simulink library "sm_robot_6legs_4bar_lib"  (R2026a)
settings: Solver=VariableStepAuto
undefined symbols (not defined in the file): frame_wid, link_h, link_th, Local, X, Z
libraries: Parts_Lib x57, sm_lib x15
Description:
  | Copyright 2018-2026 The MathWorks, Inc.
settings Model: Creator=smiller  LastModifiedBy=smiller
settings DebuggingCC: PregeneratedLibrarySubsystemCodeDiagnostic=none

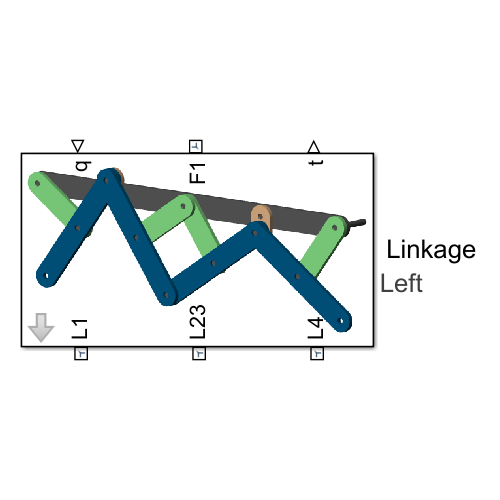
[thumbnail: Simulink's stored preview of the top-level diagram]
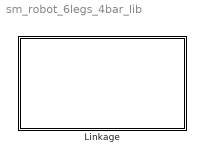
== system sm_robot_6legs_4bar_lib ==
  Linkage : Subsystem  mask(Leg Mechanism and Frame){popup_LorR=Left}
      mask prompts: popup_LorR "Side"
      mask help: Two connected four-bar linkages form three legs for one side of a 6-legged robot. Set the parameter below to select the side of the robot. Dimensions and other parameters are defined using variables in the MATLAB Workspace.
      mask init:
      | f    = Simulink.FindOptions('FollowLinks',1,'LookUnderMasks','all','regexp',1);
      | temp_rod_pth = Simulink.findBlocks(bdroot,'ReferenceBlock','.*Rod','popup_zori','.*',f);
      | 
      | if(popup_LorR == 1)
      |     rod_setting = 0;
      |     set_param([gcb '/Revolute Cam L12'],'PositionTargetValue','270');
      |     set_param([gcb '/Revolute Cam L34'],'PositionTargetValue','90');
      | else
      |     rod_setting = 1;
      |     set_param([gcb '/Revolute Cam L12'],'PositionTargetValue','90');
      |     set_param([gcb '/Revolute Cam L34'],'PositionTargetValue','270');
      | end
      | 
      | for temp_rod_i = 1:length(temp_rod_pth)
      |     set_param(temp_rod_pth(temp_rod_i),'popup_zori',rod_setting);
      | end
      settings: AttributesFormatString=%<popup_LorR>
      mask TypeOptions popup_LorR: Left | Right
      mask Display:
      | if(strcmpi(get_param(gcb,'popup_LorR'),'Left'))
      |     image('sm_robot_6legs_4bar_Linkage_Left_IMAGE.png');
      | else
      |     image('sm_robot_6legs_4bar_Linkage_Right_IMAGE.png');
      | end

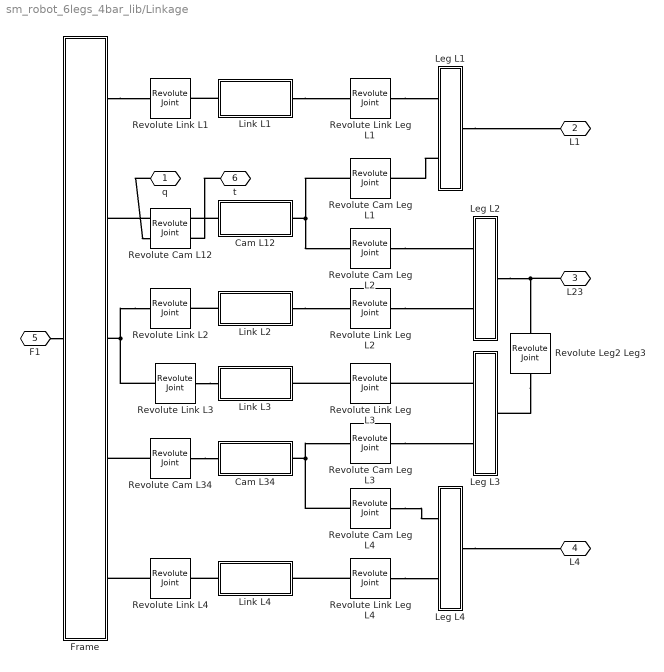
== system sm_robot_6legs_4bar_lib/Linkage ==
  Cam L12 : Subsystem
  Cam L34 : Subsystem
  Frame : Subsystem
  Leg L1 : Subsystem
  Leg L2 : Subsystem
  Leg L3 : Subsystem
  Leg L4 : Subsystem
  Link L1 : Subsystem
  Link L2 : Subsystem
  Link L3 : Subsystem
  Link L4 : Subsystem
  Revolute Leg2 Leg3 : sm_lib/Joints/Revolute Joint  JointMode=Normal  CompositeWrenchDir=FollowerOnBase  CompositeWrenchFrame=BaseFrame  SenseConstraintForce=off  SenseConstraintTorque=off  SenseTotalForce=off  SenseTotalTorque=off  PositionTargetSpecify=on  PositionTargetPriority=Low  PositionTargetValue=-90  PositionTargetValueUnits=deg  VelocityTargetSpecify=off  VelocityTargetPriority=High  VelocityTargetValue=0  VelocityTargetValueUnits=deg/s  EquilibriumPosition=0  EquilibriumPositionUnits=deg  SpringStiffness=0  SpringStiffnessUnits=N*m/deg  DampingCoefficient=0  DampingCoefficientUnits=N*m/(deg/s)  LowerLimitSpecify=off  LowerLimitBound=-90  LowerLimitBoundUnits=deg  LowerLimitStiffness=1e4  LowerLimitStiffnessUnits=N*m/deg  LowerLimitDamping=10  LowerLimitDampingUnits=N*m/(deg/s)  LowerLimitTransitionRegionWidth=0.1  LowerLimitTransitionRegionWidthUnits=deg  UpperLimitSpecify=off  UpperLimitBound=90  UpperLimitBoundUnits=deg  UpperLimitStiffness=1e4  UpperLimitStiffnessUnits=N*m/deg  UpperLimitDamping=10  UpperLimitDampingUnits=N*m/(deg/s)  UpperLimitTransitionRegionWidth=0.1  UpperLimitTransitionRegionWidthUnits=deg  TorqueActuationMode=NoTorque  MotionActuationMode=ComputedMotion  SensePosition=off  SenseVelocity=off  SenseAcceleration=off  SenseTorqueForce=off  SenseLowerLimitTorqueForce=off  SenseUpperLimitTorqueForce=off
      settings: AttributesFormatString=t0: %<PositionTargetValue> %<PositionTargetValueUnits>, %<PositionTargetPriority>
  Revolute Cam L12 : sm_lib/Joints/Revolute Joint  JointMode=Normal  CompositeWrenchDir=FollowerOnBase  CompositeWrenchFrame=BaseFrame  SenseConstraintForce=off  SenseConstraintTorque=off  SenseTotalForce=off  SenseTotalTorque=off  PositionTargetSpecify=on  PositionTargetPriority=High  PositionTargetValue=270  PositionTargetValueUnits=deg  VelocityTargetSpecify=off  VelocityTargetPriority=High  VelocityTargetValue=0  VelocityTargetValueUnits=deg/s  EquilibriumPosition=0  EquilibriumPositionUnits=deg  SpringStiffness=0  SpringStiffnessUnits=N*m/deg  DampingCoefficient=0.001  DampingCoefficientUnits=N*m/(deg/s)  LowerLimitSpecify=off  LowerLimitBound=-90  LowerLimitBoundUnits=deg  LowerLimitStiffness=1e4  LowerLimitStiffnessUnits=N*m/deg  LowerLimitDamping=10  LowerLimitDampingUnits=N*m/(deg/s)  LowerLimitTransitionRegionWidth=0.1  LowerLimitTransitionRegionWidthUnits=deg  UpperLimitSpecify=off  UpperLimitBound=90  UpperLimitBoundUnits=deg  UpperLimitStiffness=1e4  UpperLimitStiffnessUnits=N*m/deg  UpperLimitDamping=10  UpperLimitDampingUnits=N*m/(deg/s)  UpperLimitTransitionRegionWidth=0.1  UpperLimitTransitionRegionWidthUnits=deg  TorqueActuationMode=ComputedTorque  MotionActuationMode=InputMotion  SensePosition=off  SenseVelocity=off  SenseAcceleration=off  SenseTorqueForce=on  SenseLowerLimitTorqueForce=off  SenseUpperLimitTorqueForce=off
      settings: AttributesFormatString=t0: %<PositionTargetValue> %<PositionTargetValueUnits>, %<PositionTargetPriority>
  Revolute Cam L34 : sm_lib/Joints/Revolute Joint  JointMode=Normal  CompositeWrenchDir=FollowerOnBase  CompositeWrenchFrame=BaseFrame  SenseConstraintForce=off  SenseConstraintTorque=off  SenseTotalForce=off  SenseTotalTorque=off  PositionTargetSpecify=on  PositionTargetPriority=Low  PositionTargetValue=90  PositionTargetValueUnits=deg  VelocityTargetSpecify=off  VelocityTargetPriority=High  VelocityTargetValue=0  VelocityTargetValueUnits=deg/s  EquilibriumPosition=0  EquilibriumPositionUnits=deg  SpringStiffness=0  SpringStiffnessUnits=N*m/deg  DampingCoefficient=0  DampingCoefficientUnits=N*m/(deg/s)  LowerLimitSpecify=off  LowerLimitBound=-90  LowerLimitBoundUnits=deg  LowerLimitStiffness=1e4  LowerLimitStiffnessUnits=N*m/deg  LowerLimitDamping=10  LowerLimitDampingUnits=N*m/(deg/s)  LowerLimitTransitionRegionWidth=0.1  LowerLimitTransitionRegionWidthUnits=deg  UpperLimitSpecify=off  UpperLimitBound=90  UpperLimitBoundUnits=deg  UpperLimitStiffness=1e4  UpperLimitStiffnessUnits=N*m/deg  UpperLimitDamping=10  UpperLimitDampingUnits=N*m/(deg/s)  UpperLimitTransitionRegionWidth=0.1  UpperLimitTransitionRegionWidthUnits=deg  TorqueActuationMode=NoTorque  MotionActuationMode=ComputedMotion  SensePosition=off  SenseVelocity=off  SenseAcceleration=off  SenseTorqueForce=off  SenseLowerLimitTorqueForce=off  SenseUpperLimitTorqueForce=off
      settings: AttributesFormatString=t0: %<PositionTargetValue> %<PositionTargetValueUnits>, %<PositionTargetPriority>
  Revolute Cam Leg L1 : sm_lib/Joints/Revolute Joint  JointMode=Normal  CompositeWrenchDir=FollowerOnBase  CompositeWrenchFrame=BaseFrame  SenseConstraintForce=off  SenseConstraintTorque=off  SenseTotalForce=off  SenseTotalTorque=off  PositionTargetSpecify=off  PositionTargetPriority=Low  PositionTargetValue=135  PositionTargetValueUnits=deg  VelocityTargetSpecify=off  VelocityTargetPriority=High  VelocityTargetValue=0  VelocityTargetValueUnits=deg/s  EquilibriumPosition=0  EquilibriumPositionUnits=deg  SpringStiffness=0  SpringStiffnessUnits=N*m/deg  DampingCoefficient=0  DampingCoefficientUnits=N*m/(deg/s)  LowerLimitSpecify=off  LowerLimitBound=-90  LowerLimitBoundUnits=deg  LowerLimitStiffness=1e4  LowerLimitStiffnessUnits=N*m/deg  LowerLimitDamping=10  LowerLimitDampingUnits=N*m/(deg/s)  LowerLimitTransitionRegionWidth=0.1  LowerLimitTransitionRegionWidthUnits=deg  UpperLimitSpecify=off  UpperLimitBound=90  UpperLimitBoundUnits=deg  UpperLimitStiffness=1e4  UpperLimitStiffnessUnits=N*m/deg  UpperLimitDamping=10  UpperLimitDampingUnits=N*m/(deg/s)  UpperLimitTransitionRegionWidth=0.1  UpperLimitTransitionRegionWidthUnits=deg  TorqueActuationMode=NoTorque  MotionActuationMode=ComputedMotion  SensePosition=off  SenseVelocity=off  SenseAcceleration=off  SenseTorqueForce=off  SenseLowerLimitTorqueForce=off  SenseUpperLimitTorqueForce=off
  Revolute Cam Leg L2 : sm_lib/Joints/Revolute Joint  JointMode=Normal  CompositeWrenchDir=FollowerOnBase  CompositeWrenchFrame=BaseFrame  SenseConstraintForce=off  SenseConstraintTorque=off  SenseTotalForce=off  SenseTotalTorque=off  PositionTargetSpecify=off  PositionTargetPriority=Low  PositionTargetValue=-135  PositionTargetValueUnits=deg  VelocityTargetSpecify=off  VelocityTargetPriority=High  VelocityTargetValue=0  VelocityTargetValueUnits=deg/s  EquilibriumPosition=0  EquilibriumPositionUnits=deg  SpringStiffness=0  SpringStiffnessUnits=N*m/deg  DampingCoefficient=0  DampingCoefficientUnits=N*m/(deg/s)  LowerLimitSpecify=off  LowerLimitBound=-90  LowerLimitBoundUnits=deg  LowerLimitStiffness=1e4  LowerLimitStiffnessUnits=N*m/deg  LowerLimitDamping=10  LowerLimitDampingUnits=N*m/(deg/s)  LowerLimitTransitionRegionWidth=0.1  LowerLimitTransitionRegionWidthUnits=deg  UpperLimitSpecify=off  UpperLimitBound=90  UpperLimitBoundUnits=deg  UpperLimitStiffness=1e4  UpperLimitStiffnessUnits=N*m/deg  UpperLimitDamping=10  UpperLimitDampingUnits=N*m/(deg/s)  UpperLimitTransitionRegionWidth=0.1  UpperLimitTransitionRegionWidthUnits=deg  TorqueActuationMode=NoTorque  MotionActuationMode=ComputedMotion  SensePosition=off  SenseVelocity=off  SenseAcceleration=off  SenseTorqueForce=off  SenseLowerLimitTorqueForce=off  SenseUpperLimitTorqueForce=off
  Revolute Cam Leg L3 : sm_lib/Joints/Revolute Joint  JointMode=Normal  CompositeWrenchDir=FollowerOnBase  CompositeWrenchFrame=BaseFrame  SenseConstraintForce=off  SenseConstraintTorque=off  SenseTotalForce=off  SenseTotalTorque=off  PositionTargetSpecify=off  PositionTargetPriority=High  PositionTargetValue=0  PositionTargetValueUnits=deg  VelocityTargetSpecify=off  VelocityTargetPriority=High  VelocityTargetValue=0  VelocityTargetValueUnits=deg/s  EquilibriumPosition=0  EquilibriumPositionUnits=deg  SpringStiffness=0  SpringStiffnessUnits=N*m/deg  DampingCoefficient=0  DampingCoefficientUnits=N*m/(deg/s)  LowerLimitSpecify=off  LowerLimitBound=-90  LowerLimitBoundUnits=deg  LowerLimitStiffness=1e4  LowerLimitStiffnessUnits=N*m/deg  LowerLimitDamping=10  LowerLimitDampingUnits=N*m/(deg/s)  LowerLimitTransitionRegionWidth=0.1  LowerLimitTransitionRegionWidthUnits=deg  UpperLimitSpecify=off  UpperLimitBound=90  UpperLimitBoundUnits=deg  UpperLimitStiffness=1e4  UpperLimitStiffnessUnits=N*m/deg  UpperLimitDamping=10  UpperLimitDampingUnits=N*m/(deg/s)  UpperLimitTransitionRegionWidth=0.1  UpperLimitTransitionRegionWidthUnits=deg  TorqueActuationMode=NoTorque  MotionActuationMode=ComputedMotion  SensePosition=off  SenseVelocity=off  SenseAcceleration=off  SenseTorqueForce=off  SenseLowerLimitTorqueForce=off  SenseUpperLimitTorqueForce=off
  Revolute Cam Leg L4 : sm_lib/Joints/Revolute Joint  JointMode=Normal  CompositeWrenchDir=FollowerOnBase  CompositeWrenchFrame=BaseFrame  SenseConstraintForce=off  SenseConstraintTorque=off  SenseTotalForce=off  SenseTotalTorque=off  PositionTargetSpecify=off  PositionTargetPriority=High  PositionTargetValue=0  PositionTargetValueUnits=deg  VelocityTargetSpecify=off  VelocityTargetPriority=High  VelocityTargetValue=0  VelocityTargetValueUnits=deg/s  EquilibriumPosition=0  EquilibriumPositionUnits=deg  SpringStiffness=0  SpringStiffnessUnits=N*m/deg  DampingCoefficient=0  DampingCoefficientUnits=N*m/(deg/s)  LowerLimitSpecify=off  LowerLimitBound=-90  LowerLimitBoundUnits=deg  LowerLimitStiffness=1e4  LowerLimitStiffnessUnits=N*m/deg  LowerLimitDamping=10  LowerLimitDampingUnits=N*m/(deg/s)  LowerLimitTransitionRegionWidth=0.1  LowerLimitTransitionRegionWidthUnits=deg  UpperLimitSpecify=off  UpperLimitBound=90  UpperLimitBoundUnits=deg  UpperLimitStiffness=1e4  UpperLimitStiffnessUnits=N*m/deg  UpperLimitDamping=10  UpperLimitDampingUnits=N*m/(deg/s)  UpperLimitTransitionRegionWidth=0.1  UpperLimitTransitionRegionWidthUnits=deg  TorqueActuationMode=NoTorque  MotionActuationMode=ComputedMotion  SensePosition=off  SenseVelocity=off  SenseAcceleration=off  SenseTorqueForce=off  SenseLowerLimitTorqueForce=off  SenseUpperLimitTorqueForce=off
  Revolute Link L1 : sm_lib/Joints/Revolute Joint  JointMode=Normal  CompositeWrenchDir=FollowerOnBase  CompositeWrenchFrame=BaseFrame  SenseConstraintForce=off  SenseConstraintTorque=off  SenseTotalForce=off  SenseTotalTorque=off  PositionTargetSpecify=on  PositionTargetPriority=Low  PositionTargetValue=-90  PositionTargetValueUnits=deg  VelocityTargetSpecify=off  VelocityTargetPriority=High  VelocityTargetValue=0  VelocityTargetValueUnits=deg/s  EquilibriumPosition=0  EquilibriumPositionUnits=deg  SpringStiffness=0  SpringStiffnessUnits=N*m/deg  DampingCoefficient=0  DampingCoefficientUnits=N*m/(deg/s)  LowerLimitSpecify=off  LowerLimitBound=-90  LowerLimitBoundUnits=deg  LowerLimitStiffness=1e4  LowerLimitStiffnessUnits=N*m/deg  LowerLimitDamping=10  LowerLimitDampingUnits=N*m/(deg/s)  LowerLimitTransitionRegionWidth=0.1  LowerLimitTransitionRegionWidthUnits=deg  UpperLimitSpecify=off  UpperLimitBound=90  UpperLimitBoundUnits=deg  UpperLimitStiffness=1e4  UpperLimitStiffnessUnits=N*m/deg  UpperLimitDamping=10  UpperLimitDampingUnits=N*m/(deg/s)  UpperLimitTransitionRegionWidth=0.1  UpperLimitTransitionRegionWidthUnits=deg  TorqueActuationMode=NoTorque  MotionActuationMode=ComputedMotion  SensePosition=off  SenseVelocity=off  SenseAcceleration=off  SenseTorqueForce=off  SenseLowerLimitTorqueForce=off  SenseUpperLimitTorqueForce=off
      settings: AttributesFormatString=t0: %<PositionTargetValue> %<PositionTargetValueUnits>, %<PositionTargetPriority>
  Revolute Link L2 : sm_lib/Joints/Revolute Joint  JointMode=Normal  CompositeWrenchDir=FollowerOnBase  CompositeWrenchFrame=BaseFrame  SenseConstraintForce=off  SenseConstraintTorque=off  SenseTotalForce=off  SenseTotalTorque=off  PositionTargetSpecify=off  PositionTargetPriority=High  PositionTargetValue=0  PositionTargetValueUnits=deg  VelocityTargetSpecify=off  VelocityTargetPriority=High  VelocityTargetValue=0  VelocityTargetValueUnits=deg/s  EquilibriumPosition=0  EquilibriumPositionUnits=deg  SpringStiffness=0  SpringStiffnessUnits=N*m/deg  DampingCoefficient=0  DampingCoefficientUnits=N*m/(deg/s)  LowerLimitSpecify=off  LowerLimitBound=-90  LowerLimitBoundUnits=deg  LowerLimitStiffness=1e4  LowerLimitStiffnessUnits=N*m/deg  LowerLimitDamping=10  LowerLimitDampingUnits=N*m/(deg/s)  LowerLimitTransitionRegionWidth=0.1  LowerLimitTransitionRegionWidthUnits=deg  UpperLimitSpecify=off  UpperLimitBound=90  UpperLimitBoundUnits=deg  UpperLimitStiffness=1e4  UpperLimitStiffnessUnits=N*m/deg  UpperLimitDamping=10  UpperLimitDampingUnits=N*m/(deg/s)  UpperLimitTransitionRegionWidth=0.1  UpperLimitTransitionRegionWidthUnits=deg  TorqueActuationMode=NoTorque  MotionActuationMode=ComputedMotion  SensePosition=off  SenseVelocity=off  SenseAcceleration=off  SenseTorqueForce=off  SenseLowerLimitTorqueForce=off  SenseUpperLimitTorqueForce=off
  Revolute Link L3 : sm_lib/Joints/Revolute Joint  JointMode=Normal  CompositeWrenchDir=FollowerOnBase  CompositeWrenchFrame=BaseFrame  SenseConstraintForce=off  SenseConstraintTorque=off  SenseTotalForce=off  SenseTotalTorque=off  PositionTargetSpecify=off  PositionTargetPriority=Low  PositionTargetValue=-135  PositionTargetValueUnits=deg  VelocityTargetSpecify=off  VelocityTargetPriority=High  VelocityTargetValue=0  VelocityTargetValueUnits=deg/s  EquilibriumPosition=0  EquilibriumPositionUnits=deg  SpringStiffness=0  SpringStiffnessUnits=N*m/deg  DampingCoefficient=0  DampingCoefficientUnits=N*m/(deg/s)  LowerLimitSpecify=off  LowerLimitBound=-90  LowerLimitBoundUnits=deg  LowerLimitStiffness=1e4  LowerLimitStiffnessUnits=N*m/deg  LowerLimitDamping=10  LowerLimitDampingUnits=N*m/(deg/s)  LowerLimitTransitionRegionWidth=0.1  LowerLimitTransitionRegionWidthUnits=deg  UpperLimitSpecify=off  UpperLimitBound=90  UpperLimitBoundUnits=deg  UpperLimitStiffness=1e4  UpperLimitStiffnessUnits=N*m/deg  UpperLimitDamping=10  UpperLimitDampingUnits=N*m/(deg/s)  UpperLimitTransitionRegionWidth=0.1  UpperLimitTransitionRegionWidthUnits=deg  TorqueActuationMode=NoTorque  MotionActuationMode=ComputedMotion  SensePosition=off  SenseVelocity=off  SenseAcceleration=off  SenseTorqueForce=off  SenseLowerLimitTorqueForce=off  SenseUpperLimitTorqueForce=off
  Revolute Link L4 : sm_lib/Joints/Revolute Joint  JointMode=Normal  CompositeWrenchDir=FollowerOnBase  CompositeWrenchFrame=BaseFrame  SenseConstraintForce=off  SenseConstraintTorque=off  SenseTotalForce=off  SenseTotalTorque=off  PositionTargetSpecify=on  PositionTargetPriority=Low  PositionTargetValue=-90  PositionTargetValueUnits=deg  VelocityTargetSpecify=off  VelocityTargetPriority=High  VelocityTargetValue=0  VelocityTargetValueUnits=deg/s  EquilibriumPosition=0  EquilibriumPositionUnits=deg  SpringStiffness=0  SpringStiffnessUnits=N*m/deg  DampingCoefficient=0  DampingCoefficientUnits=N*m/(deg/s)  LowerLimitSpecify=off  LowerLimitBound=-90  LowerLimitBoundUnits=deg  LowerLimitStiffness=1e4  LowerLimitStiffnessUnits=N*m/deg  LowerLimitDamping=10  LowerLimitDampingUnits=N*m/(deg/s)  LowerLimitTransitionRegionWidth=0.1  LowerLimitTransitionRegionWidthUnits=deg  UpperLimitSpecify=off  UpperLimitBound=90  UpperLimitBoundUnits=deg  UpperLimitStiffness=1e4  UpperLimitStiffnessUnits=N*m/deg  UpperLimitDamping=10  UpperLimitDampingUnits=N*m/(deg/s)  UpperLimitTransitionRegionWidth=0.1  UpperLimitTransitionRegionWidthUnits=deg  TorqueActuationMode=NoTorque  MotionActuationMode=ComputedMotion  SensePosition=off  SenseVelocity=off  SenseAcceleration=off  SenseTorqueForce=off  SenseLowerLimitTorqueForce=off  SenseUpperLimitTorqueForce=off
      settings: AttributesFormatString=t0: %<PositionTargetValue> %<PositionTargetValueUnits>, %<PositionTargetPriority>
  Revolute Link Leg L{1..4} (4 alike) : sm_lib/Joints/Revolute Joint  JointMode=Normal  CompositeWrenchDir=FollowerOnBase  CompositeWrenchFrame=BaseFrame  SenseConstraintForce=off  SenseConstraintTorque=off  SenseTotalForce=off  SenseTotalTorque=off  PositionTargetSpecify=off  PositionTargetPriority=High  PositionTargetValue=0  PositionTargetValueUnits=deg  VelocityTargetSpecify=off  VelocityTargetPriority=High  VelocityTargetValue=0  VelocityTargetValueUnits=deg/s  EquilibriumPosition=0  EquilibriumPositionUnits=deg  SpringStiffness=0  SpringStiffnessUnits=N*m/deg  DampingCoefficient=0  DampingCoefficientUnits=N*m/(deg/s)  LowerLimitSpecify=off  LowerLimitBound=-90  LowerLimitBoundUnits=deg  LowerLimitStiffness=1e4  LowerLimitStiffnessUnits=N*m/deg  LowerLimitDamping=10  LowerLimitDampingUnits=N*m/(deg/s)  LowerLimitTransitionRegionWidth=0.1  LowerLimitTransitionRegionWidthUnits=deg  UpperLimitSpecify=off  UpperLimitBound=90  UpperLimitBoundUnits=deg  UpperLimitStiffness=1e4  UpperLimitStiffnessUnits=N*m/deg  UpperLimitDamping=10  UpperLimitDampingUnits=N*m/(deg/s)  UpperLimitTransitionRegionWidth=0.1  UpperLimitTransitionRegionWidthUnits=deg  TorqueActuationMode=NoTorque  MotionActuationMode=ComputedMotion  SensePosition=off  SenseVelocity=off  SenseAcceleration=off  SenseTorqueForce=off  SenseLowerLimitTorqueForce=off  SenseUpperLimitTorqueForce=off
  q : PMIOPort  Side=Left
  L1 : PMIOPort  Port=2  Side=Right
  L23 : PMIOPort  Port=3  Side=Right
  L4 : PMIOPort  Port=4  Side=Right
  F1 : PMIOPort  Port=5  Side=Left
  t : PMIOPort  Port=6  Side=Left
  connections:
  F1/RConn1 -- Frame/RConn1
  Cam L12/RConn1 -- Revolute Cam L12/RConn1
  Leg L4/RConn1 -- L4/RConn1
  Leg L1/LConn2 -- Revolute Cam Leg L1/RConn1
  Leg L2/RConn1 -- L23/RConn1 -- Revolute Leg2 Leg3/LConn1
  Link L2/RConn1 -- Revolute Link Leg L2/RConn1
  Revolute Link L2/LConn1 -- Frame/LConn3 -- Revolute Link L3/LConn1
  Revolute Cam Leg L4/LConn1 -- Revolute Cam Leg L3/LConn1 -- Cam L34/RConn1
  Revolute Leg2 Leg3/RConn1 -- Leg L3/RConn1
  Leg L3/LConn1 -- Revolute Link Leg L3/RConn1
  Revolute Cam L34/RConn1 -- Cam L34/LConn1
  Link L4/LConn1 -- Revolute Link L4/RConn1
  Frame/LConn1 -- Revolute Link L1/LConn1
  Revolute Link Leg L2/LConn1 -- Leg L2/LConn2
  Revolute Cam L12/LConn1 -- Frame/LConn2
  Revolute Cam Leg L2/RConn1 -- Leg L2/LConn1
  Revolute Cam L34/LConn1 -- Frame/LConn4
  Revolute Cam Leg L3/RConn1 -- Leg L3/LConn2
  Revolute Cam Leg L4/RConn1 -- Leg L4/LConn1
  Revolute Link Leg L4/RConn1 -- Leg L4/LConn2
  Revolute Link Leg L3/LConn1 -- Link L3/LConn1
  Link L2/LConn1 -- Revolute Link L2/RConn1
  Link L1/LConn1 -- Revolute Link Leg L1/LConn1
  Cam L12/LConn1 -- Revolute Cam Leg L2/LConn1 -- Revolute Cam Leg L1/LConn1
  Revolute Link Leg L4/LConn1 -- Link L4/RConn1
  Revolute Link Leg L1/RConn1 -- Leg L1/LConn1
  Revolute Link L4/LConn1 -- Frame/LConn5
  Link L1/RConn1 -- Revolute Link L1/RConn1
  Leg L1/RConn1 -- L1/RConn1
  q/RConn1 -- Revolute Cam L12/LConn2
  Revolute Link L3/RConn1 -- Link L3/RConn1
  t/RConn1 -- Revolute Cam L12/RConn2

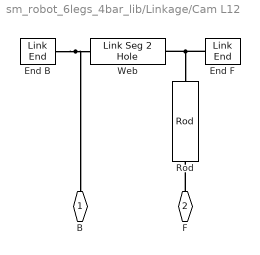
== system sm_robot_6legs_4bar_lib/Linkage/Cam L12 ==
  End B : Parts_Lib/Link End  circ_radout=link_h/2  circ_radin=rad_hole  popup_holelr=-X  deg_1=90  deg_2=270  circ_len=link_th  circ_rho=part_rho  circ_color=cam_clr  circ_opc=1
  End F : Parts_Lib/Link End  circ_radout=link_h/2  circ_radin=rad_hole  popup_holelr=+X  deg_1=-90  deg_2=90  circ_len=link_th  circ_rho=part_rho  circ_color=cam_clr  circ_opc=1
  Rod : Parts_Lib/Rod  rod_rad=rad_hole  rod_len=link_th  rod_rho=part_rho  rod_color=pin_clr  popup_zori=Local +Z  popup_markings=None  mark_radius_range=[0.5 1.01]  mark_length_range=1.005  mark_angle_range=30  mark_color=[1 1 1]
  Web : Parts_Lib/Link Seg 2 Hole  link_len=cam_l  link_width=link_h  link_radh=rad_hole  link_thickness=link_th  link_rho=part_rho  link_color=cam_clr  link_opc=1
  B : PMIOPort  Side=Right
  F : PMIOPort  Port=2  Side=Left
  connections:
  End B/LConn1 -- B/RConn1 -- Web/LConn1
  End F/LConn1 -- Web/RConn1 -- Rod/RConn1
  F/RConn1 -- Rod/LConn1

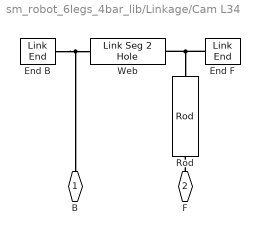
== system sm_robot_6legs_4bar_lib/Linkage/Cam L34 ==
  End B : Parts_Lib/Link End  circ_radout=link_h/2  circ_radin=rad_hole  popup_holelr=-X  deg_1=90  deg_2=270  circ_len=link_th  circ_rho=part_rho  circ_color=cam_clr  circ_opc=1
  End F : Parts_Lib/Link End  circ_radout=link_h/2  circ_radin=rad_hole  popup_holelr=+X  deg_1=-90  deg_2=90  circ_len=link_th  circ_rho=part_rho  circ_color=cam_clr  circ_opc=1
  Rod : Parts_Lib/Rod  rod_rad=rad_hole  rod_len=link_th  rod_rho=part_rho  rod_color=pin_clr  popup_zori=Local +Z  popup_markings=None  mark_radius_range=[0.5 1.01]  mark_length_range=1.005  mark_angle_range=30  mark_color=[1 1 1]
  Web : Parts_Lib/Link Seg 2 Hole  link_len=cam_l  link_width=link_h  link_radh=rad_hole  link_thickness=link_th  link_rho=part_rho  link_color=cam_clr  link_opc=1
  B : PMIOPort  Side=Left
  F : PMIOPort  Port=2  Side=Right
  connections:
  End F/LConn1 -- Web/RConn1 -- Rod/RConn1
  F/RConn1 -- Rod/LConn1
  Web/LConn1 -- End B/LConn1 -- B/RConn1

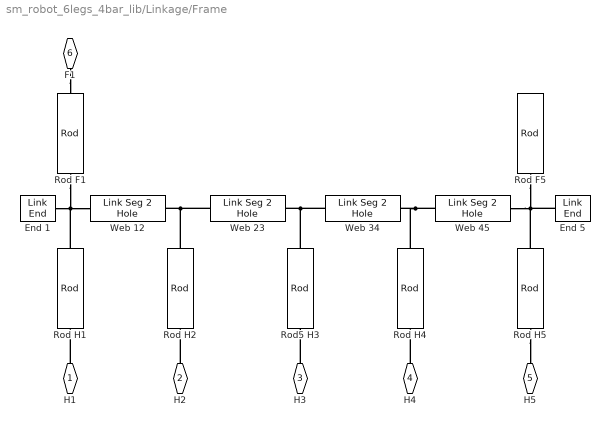
== system sm_robot_6legs_4bar_lib/Linkage/Frame ==
  End 1 : Parts_Lib/Link End  circ_radout=link_h/2  circ_radin=rad_hole  popup_holelr=-X  deg_1=90  deg_2=270  circ_len=link_th  circ_rho=part_rho  circ_color=fra_clr  circ_opc=1
  End 5 : Parts_Lib/Link End  circ_radout=link_h/2  circ_radin=rad_hole  popup_holelr=+X  deg_1=-90  deg_2=90  circ_len=link_th  circ_rho=part_rho  circ_color=fra_clr  circ_opc=1
  Rod F1 : Parts_Lib/Rod  rod_rad=rad_hole  rod_len=frame_wid/2  rod_rho=part_rho  rod_color=pin_clr  popup_zori=Local +Z  popup_markings=None  mark_radius_range=[0.5 1.01]  mark_length_range=1.005  mark_angle_range=30  mark_color=[1 1 1]
  Rod F5 : Parts_Lib/Rod  rod_rad=rad_hole  rod_len=frame_wid/2  rod_rho=part_rho  rod_color=pin_clr  popup_zori=Local +Z  popup_markings=None  mark_radius_range=[0.5 1.01]  mark_length_range=1.005  mark_angle_range=30  mark_color=[1 1 1]
  Rod H{1..2,4..5} (4 alike) : Parts_Lib/Rod  rod_rad=rad_hole  rod_len=link_th  rod_rho=part_rho  rod_color=pin_clr  popup_zori=Local +Z  popup_markings=None  mark_radius_range=[0.5 1.01]  mark_length_range=1.005  mark_angle_range=30  mark_color=[1 1 1]
  Rod5 H3 : Parts_Lib/Rod  rod_rad=rad_hole  rod_len=link_th  rod_rho=part_rho  rod_color=pin_clr  popup_zori=Local +Z  popup_markings=None  mark_radius_range=[0.5 1.01]  mark_length_range=1.005  mark_angle_range=30  mark_color=[1 1 1]
  Web {12,23,34,45} (4 alike) : Parts_Lib/Link Seg 2 Hole  link_len=frame_xhole  link_width=link_h  link_radh=rad_hole  link_thickness=link_th  link_rho=part_rho  link_color=fra_clr  link_opc=1
  H1 : PMIOPort  Side=Left
  H2 : PMIOPort  Port=2  Side=Left
  H3 : PMIOPort  Port=3  Side=Left
  H4 : PMIOPort  Port=4  Side=Left
  H5 : PMIOPort  Port=5  Side=Left
  F1 : PMIOPort  Port=6  Side=Right
  connections:
  Web 23/LConn1 -- Rod H2/RConn1 -- Web 12/RConn1
  End 5/LConn1 -- Rod F5/LConn1 -- Rod H5/RConn1 -- Web 45/RConn1
  End 1/LConn1 -- Rod F1/LConn1 -- Rod H1/RConn1 -- Web 12/LConn1
  Web 45/LConn1 -- Rod H4/RConn1 -- Web 34/RConn1
  Web 34/LConn1 -- Rod5 H3/RConn1 -- Web 23/RConn1
  Rod H5/LConn1 -- H5/RConn1
  H4/RConn1 -- Rod H4/LConn1
  H3/RConn1 -- Rod5 H3/LConn1
  H2/RConn1 -- Rod H2/LConn1
  H1/RConn1 -- Rod H1/LConn1
  F1/RConn1 -- Rod F1/RConn1

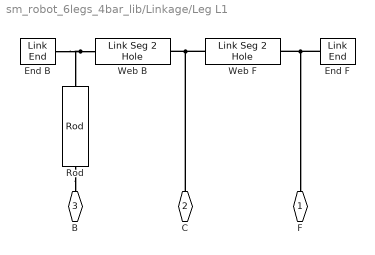
== system sm_robot_6legs_4bar_lib/Linkage/Leg L1 ==
  End B : Parts_Lib/Link End  circ_radout=link_h/2  circ_radin=rad_hole  popup_holelr=-X  deg_1=90  deg_2=270  circ_len=link_th  circ_rho=part_rho  circ_color=leg_clr  circ_opc=1
  End F : Parts_Lib/Link End  circ_radout=link_h/2  circ_radin=rad_hole  popup_holelr=+X  deg_1=-90  deg_2=90  circ_len=link_th  circ_rho=part_rho  circ_color=leg_clr  circ_opc=1
  Rod : Parts_Lib/Rod  rod_rad=rad_hole  rod_len=link_th  rod_rho=part_rho  rod_color=pin_clr  popup_zori=Local +Z  popup_markings=None  mark_radius_range=[0.5 1.01]  mark_length_range=1.005  mark_angle_range=30  mark_color=[1 1 1]
  Web B : Parts_Lib/Link Seg 2 Hole  link_len=fol_l  link_width=link_h  link_radh=rad_hole  link_thickness=link_th  link_rho=part_rho  link_color=leg_clr  link_opc=1
  Web F : Parts_Lib/Link Seg 2 Hole  link_len=fol_l  link_width=link_h  link_radh=rad_hole  link_thickness=link_th  link_rho=part_rho  link_color=leg_clr  link_opc=1
  F : PMIOPort  Side=Right
  C : PMIOPort  Port=2  Side=Left
  B : PMIOPort  Port=3  Side=Left
  connections:
  Rod/RConn1 -- B/RConn1
  Web B/LConn1 -- Rod/LConn1 -- End B/LConn1
  End F/LConn1 -- F/RConn1 -- Web F/RConn1
  Web F/LConn1 -- C/RConn1 -- Web B/RConn1

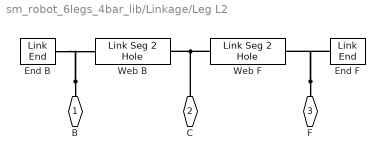
== system sm_robot_6legs_4bar_lib/Linkage/Leg L2 ==
  End B : Parts_Lib/Link End  circ_radout=link_h/2  circ_radin=rad_hole  popup_holelr=-X  deg_1=90  deg_2=270  circ_len=link_th  circ_rho=part_rho  circ_color=leg_clr  circ_opc=1
  End F : Parts_Lib/Link End  circ_radout=link_h/2  circ_radin=rad_hole  popup_holelr=+X  deg_1=-90  deg_2=90  circ_len=link_th  circ_rho=part_rho  circ_color=leg_clr  circ_opc=1
  Web B : Parts_Lib/Link Seg 2 Hole  link_len=fol_l  link_width=link_h  link_radh=rad_hole  link_thickness=link_th  link_rho=part_rho  link_color=leg_clr  link_opc=1
  Web F : Parts_Lib/Link Seg 2 Hole  link_len=fol_l  link_width=link_h  link_radh=rad_hole  link_thickness=link_th  link_rho=part_rho  link_color=leg_clr  link_opc=1
  B : PMIOPort  Side=Left
  C : PMIOPort  Port=2  Side=Left
  F : PMIOPort  Port=3  Side=Right
  connections:
  B/RConn1 -- End B/LConn1 -- Web B/LConn1
  F/RConn1 -- Web F/RConn1 -- End F/LConn1
  Web F/LConn1 -- Web B/RConn1 -- C/RConn1

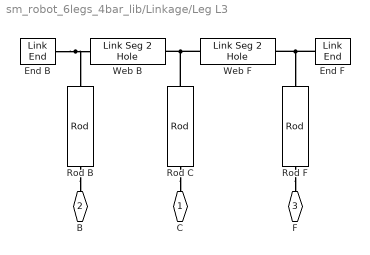
== system sm_robot_6legs_4bar_lib/Linkage/Leg L3 ==
  End B : Parts_Lib/Link End  circ_radout=link_h/2  circ_radin=rad_hole  popup_holelr=-X  deg_1=90  deg_2=270  circ_len=link_th  circ_rho=part_rho  circ_color=leg_clr  circ_opc=1
  End F : Parts_Lib/Link End  circ_radout=link_h/2  circ_radin=rad_hole  popup_holelr=+X  deg_1=-90  deg_2=90  circ_len=link_th  circ_rho=part_rho  circ_color=leg_clr  circ_opc=1
  Rod B : Parts_Lib/Rod  rod_rad=rad_hole  rod_len=link_th  rod_rho=part_rho  rod_color=pin_clr  popup_zori=Local +Z  popup_markings=None  mark_radius_range=[0.5 1.01]  mark_length_range=1.005  mark_angle_range=30  mark_color=[1 1 1]
  Rod C : Parts_Lib/Rod  rod_rad=rad_hole  rod_len=link_th  rod_rho=part_rho  rod_color=pin_clr  popup_zori=Local +Z  popup_markings=None  mark_radius_range=[0.5 1.01]  mark_length_range=1.005  mark_angle_range=30  mark_color=[1 1 1]
  Rod F : Parts_Lib/Rod  rod_rad=rad_hole  rod_len=link_th  rod_rho=part_rho  rod_color=pin_clr  popup_zori=Local +Z  popup_markings=None  mark_radius_range=[0.5 1.01]  mark_length_range=1.005  mark_angle_range=30  mark_color=[1 1 1]
  Web B : Parts_Lib/Link Seg 2 Hole  link_len=fol_l  link_width=link_h  link_radh=rad_hole  link_thickness=link_th  link_rho=part_rho  link_color=leg_clr  link_opc=1
  Web F : Parts_Lib/Link Seg 2 Hole  link_len=fol_l  link_width=link_h  link_radh=rad_hole  link_thickness=link_th  link_rho=part_rho  link_color=leg_clr  link_opc=1
  C : PMIOPort  Side=Left
  B : PMIOPort  Port=2  Side=Left
  F : PMIOPort  Port=3  Side=Right
  connections:
  Web F/LConn1 -- Web B/RConn1 -- Rod C/LConn1
  End F/LConn1 -- Web F/RConn1 -- Rod F/LConn1
  Rod B/RConn1 -- B/RConn1
  End B/LConn1 -- Web B/LConn1 -- Rod B/LConn1
  Rod C/RConn1 -- C/RConn1
  Rod F/RConn1 -- F/RConn1

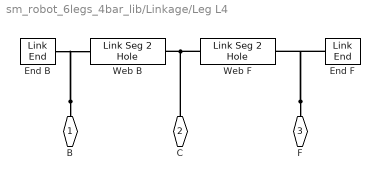
== system sm_robot_6legs_4bar_lib/Linkage/Leg L4 ==
  End B : Parts_Lib/Link End  circ_radout=link_h/2  circ_radin=rad_hole  popup_holelr=-X  deg_1=90  deg_2=270  circ_len=link_th  circ_rho=part_rho  circ_color=leg_clr  circ_opc=1
  End F : Parts_Lib/Link End  circ_radout=link_h/2  circ_radin=rad_hole  popup_holelr=+X  deg_1=-90  deg_2=90  circ_len=link_th  circ_rho=part_rho  circ_color=leg_clr  circ_opc=1
  Web B : Parts_Lib/Link Seg 2 Hole  link_len=fol_l  link_width=link_h  link_radh=rad_hole  link_thickness=link_th  link_rho=part_rho  link_color=leg_clr  link_opc=1
  Web F : Parts_Lib/Link Seg 2 Hole  link_len=fol_l  link_width=link_h  link_radh=rad_hole  link_thickness=link_th  link_rho=part_rho  link_color=leg_clr  link_opc=1
  B : PMIOPort  Side=Left
  C : PMIOPort  Port=2  Side=Left
  F : PMIOPort  Port=3  Side=Right
  connections:
  B/RConn1 -- Web B/LConn1 -- End B/LConn1
  F/RConn1 -- End F/LConn1 -- Web F/RConn1
  Web F/LConn1 -- C/RConn1 -- Web B/RConn1

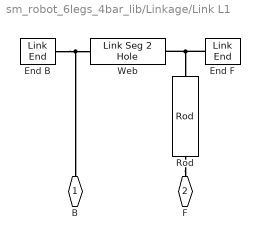
== system sm_robot_6legs_4bar_lib/Linkage/Link L1 ==
  End B : Parts_Lib/Link End  circ_radout=link_h/2  circ_radin=rad_hole  popup_holelr=-X  deg_1=90  deg_2=270  circ_len=link_th  circ_rho=part_rho  circ_color=fol_clr  circ_opc=1
  End F : Parts_Lib/Link End  circ_radout=link_h/2  circ_radin=rad_hole  popup_holelr=+X  deg_1=-90  deg_2=90  circ_len=link_th  circ_rho=part_rho  circ_color=fol_clr  circ_opc=1
  Rod : Parts_Lib/Rod  rod_rad=rad_hole  rod_len=link_th*2  rod_rho=part_rho  rod_color=pin_clr  popup_zori=Local +Z  popup_markings=None  mark_radius_range=[0.5 1.01]  mark_length_range=1.005  mark_angle_range=30  mark_color=[1 1 1]
  Web : Parts_Lib/Link Seg 2 Hole  link_len=fol_l  link_width=link_h  link_radh=rad_hole  link_thickness=link_th  link_rho=part_rho  link_color=fol_clr  link_opc=1
  B : PMIOPort  Side=Right
  F : PMIOPort  Port=2  Side=Left
  connections:
  End F/LConn1 -- Web/RConn1 -- Rod/RConn1
  Rod/LConn1 -- F/RConn1
  End B/LConn1 -- B/RConn1 -- Web/LConn1

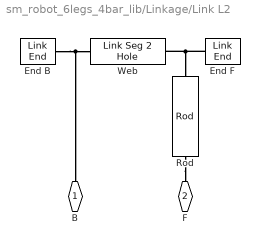
== system sm_robot_6legs_4bar_lib/Linkage/Link L2 ==
  End B : Parts_Lib/Link End  circ_radout=link_h/2  circ_radin=rad_hole  popup_holelr=-X  deg_1=90  deg_2=270  circ_len=link_th  circ_rho=part_rho  circ_color=fol_clr  circ_opc=1
  End F : Parts_Lib/Link End  circ_radout=link_h/2  circ_radin=rad_hole  popup_holelr=+X  deg_1=-90  deg_2=90  circ_len=link_th  circ_rho=part_rho  circ_color=fol_clr  circ_opc=1
  Rod : Parts_Lib/Rod  rod_rad=rad_hole  rod_len=link_th  rod_rho=part_rho  rod_color=pin_clr  popup_zori=Local +Z  popup_markings=None  mark_radius_range=[0.5 1.01]  mark_length_range=1.005  mark_angle_range=30  mark_color=[1 1 1]
  Web : Parts_Lib/Link Seg 2 Hole  link_len=fol_l  link_width=link_h  link_radh=rad_hole  link_thickness=link_th  link_rho=part_rho  link_color=fol_clr  link_opc=1
  B : PMIOPort  Side=Left
  F : PMIOPort  Port=2  Side=Right
  connections:
  End F/LConn1 -- Web/RConn1 -- Rod/RConn1
  End B/LConn1 -- B/RConn1 -- Web/LConn1
  Rod/LConn1 -- F/RConn1

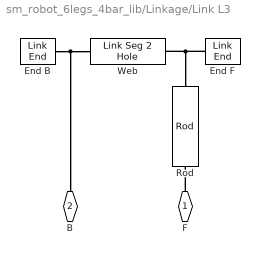
== system sm_robot_6legs_4bar_lib/Linkage/Link L3 ==
  End B : Parts_Lib/Link End  circ_radout=link_h/2  circ_radin=rad_hole  popup_holelr=-X  deg_1=90  deg_2=270  circ_len=link_th  circ_rho=part_rho  circ_color=fol_clr  circ_opc=1
  End F : Parts_Lib/Link End  circ_radout=link_h/2  circ_radin=rad_hole  popup_holelr=+X  deg_1=-90  deg_2=90  circ_len=link_th  circ_rho=part_rho  circ_color=fol_clr  circ_opc=1
  Rod : Parts_Lib/Rod  rod_rad=rad_hole  rod_len=link_th  rod_rho=part_rho  rod_color=pin_clr  popup_zori=Local +Z  popup_markings=None  mark_radius_range=[0.5 1.01]  mark_length_range=1.005  mark_angle_range=30  mark_color=[1 1 1]
  Web : Parts_Lib/Link Seg 2 Hole  link_len=fol_l  link_width=link_h  link_radh=rad_hole  link_thickness=link_th  link_rho=part_rho  link_color=fol_clr  link_opc=1
  F : PMIOPort  Side=Right
  B : PMIOPort  Port=2  Side=Left
  connections:
  End F/LConn1 -- Web/RConn1 -- Rod/LConn1
  F/RConn1 -- Rod/RConn1
  End B/LConn1 -- Web/LConn1 -- B/RConn1

== system sm_robot_6legs_4bar_lib/Linkage/Link L4 ==
  End B : Parts_Lib/Link End  circ_radout=link_h/2  circ_radin=rad_hole  popup_holelr=-X  deg_1=90  deg_2=270  circ_len=link_th  circ_rho=part_rho  circ_color=fol_clr  circ_opc=1
  End F : Parts_Lib/Link End  circ_radout=link_h/2  circ_radin=rad_hole  popup_holelr=+X  deg_1=-90  deg_2=90  circ_len=link_th  circ_rho=part_rho  circ_color=fol_clr  circ_opc=1
  Rod : Parts_Lib/Rod  rod_rad=rad_hole  rod_len=link_th  rod_rho=part_rho  rod_color=pin_clr  popup_zori=Local +Z  popup_markings=None  mark_radius_range=[0.5 1.01]  mark_length_range=1.005  mark_angle_range=30  mark_color=[1 1 1]
  Web : Parts_Lib/Link Seg 2 Hole  link_len=fol_l  link_width=link_h  link_radh=rad_hole  link_thickness=link_th  link_rho=part_rho  link_color=fol_clr  link_opc=1
  B : PMIOPort  Side=Left
  F : PMIOPort  Port=2  Side=Right
  connections:
  End F/LConn1 -- Web/RConn1 -- Rod/RConn1
  End B/LConn1 -- B/RConn1 -- Web/LConn1
  F/RConn1 -- Rod/LConn1
